simulink model "uebertragungsFunktion"  (R2017b)
settings: Solver=ode8  StartTime=0.0  StopTime=t_max  FixedStep=stepSize  RelTol=1e-3
values from neighbouring files (symbols this model uses):
  c = 10    [Aufgabe2_parameterInit.m]
  d = .5    (= 0.5)    [Aufgabe2_parameterInit.m]
  m = 1    [Aufgabe2_parameterInit.m]
undefined symbols (not defined in the file or in its folder): omega
settings Model: Creator=jens  LastModifiedBy=jens

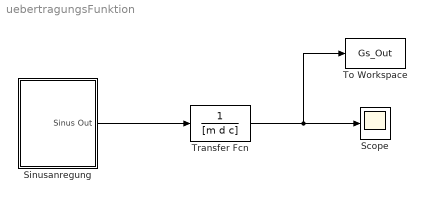
== system uebertragungsFunktion ==
  Scope : Scope
  Sinusanregung : Subsystem
  To Workspace : ToWorkspace  VariableName=Gs_Out  SampleTime=-1
  Transfer Fcn : TransferFcn  Denominator=[m d c]
  wires:
  Sinusanregung/1(Sinus Out) -> Transfer Fcn/1
  Transfer Fcn/1 -> To Workspace/1, Scope/1

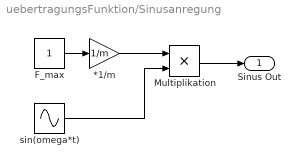
== system uebertragungsFunktion/Sinusanregung ==
  *1/m : Gain  Gain=1/m
  F_max : Constant
  Multiplikation : Product
  sin(omega*t) : Sin  Frequency=omega  SampleTime=0
  Sinus Out : Outport
  wires:
  sin(omega*t)/1 -> Multiplikation/2
  *1/m/1 -> Multiplikation/1
  Multiplikation/1 -> Sinus Out/1
  F_max/1 -> *1/m/1
